simulink model "MotorModelContinuos"  (R2019b)
settings: Solver=VariableStepAuto  StartTime=0.0  StopTime=10  RelTol=1e-3
undefined symbols (not defined in the file or in its folder): C_max, I, I_max, J_m_star, k_t, L, P, R, tau_e, Ts
libraries: simulink x1
settings Model: Creator=AndreaCalegari  LastModifiedBy=AndreaCalegari

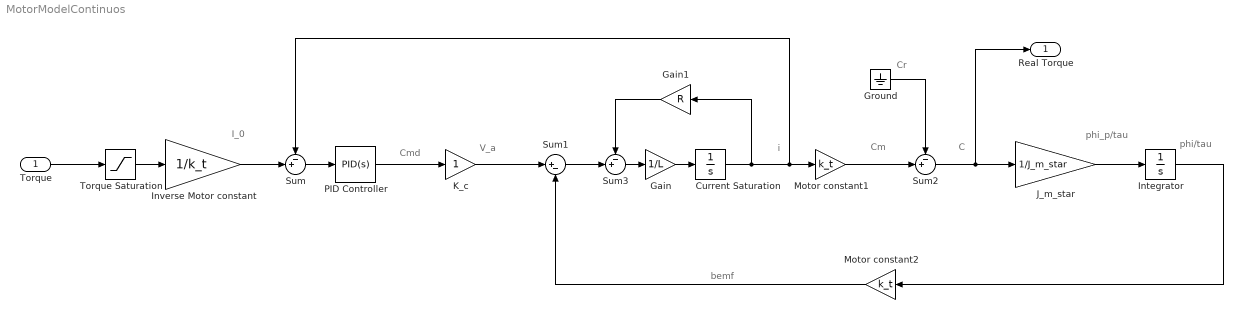
== system MotorModelContinuos ==
  note: i
  note: phi_p/tau
  note: I_0
  note: Cr
  note: bemf
  note: V_a
  note: C
  note: phi/tau
  note: Cmd
  note: Cm
  Torque : Inport  SampleTime=Ts
  Current Saturation : Integrator  LimitOutput=on  UpperSaturationLimit=I_max  LowerSaturationLimit=-I_max
  Gain : Gain  Gain=1/L
  Gain1 : Gain  Gain=R
  Ground : Ground
  Integrator : Integrator
  Inverse Motor constant : Gain  Gain=1/k_t
  "J_m_star " : Gain  Gain=1/J_m_star
  K_c : Gain
  Motor constant1 : Gain  Gain=k_t
  Motor constant2 : Gain  Gain=k_t
  PID Controller : simulink/Continuous/PID Controller  Controller=PID  Form=Parallel  TimeDomain=Continuous-time  SampleTime=-1  IntegratorMethod=Forward Euler  FilterMethod=Forward Euler  ControllerParametersSource=internal  P=P  I=I  D=0  UseFilter=on  N=100  TunerSelectOption=Transfer Function Based (PID Tuner App)  InitialConditionSource=internal  InitialConditionForIntegrator=0  InitialConditionForFilter=0  DifferentiatorICPrevScaledInput=0  ExternalReset=none  TrackingMode=off  Kt=1/tau_e  LimitOutput=off  UpperSaturationLimit=400  LowerSaturationLimit=-400  LinearizeAsGain=off  AntiWindupMode=clamping  Kb=1  POutMin=[]  POutMax=[]  IOutMin=[]  IOutMax=[]  DOutMin=[]  DOutMax=[]  NOutMin=[]  NOutMax=[]  SumOutMin=[]  SumOutMax=[]  SaturationOutMin=[]  SaturationOutMax=[]  PParamMin=[]  PParamMax=[]  IParamMin=[]  IParamMax=[]  DParamMin=[]  DParamMax=[]  NParamMin=[]  NParamMax=[]  KbParamMin=[]  KbParamMax=[]  KtParamMin=[]  KtParamMax=[]  KbOutMin=[]  KbOutMax=[]  KtOutMin=[]  KtOutMax=[]  IntegratorOutMin=[]  IntegratorOutMax=[]  FilterOutMin=[]  FilterOutMax=[]  SumI1OutMin=[]  SumI1OutMax=[]  SumI2OutMin=[]  SumI2OutMax=[]  SumI3OutMin=[]  SumI3OutMax=[]  SumI4OutMin=[]  SumI4OutMax=[]  SumDOutMin=[]  SumDOutMax=[]  DifferentiatorOutMin=[]  DifferentiatorOutMax=[]  FilterDiffOutCoefMin=[]  FilterDiffOutCoefMax=[]  ReciprocalOutMin=[]  ReciprocalOutMax=[]  SumDenOutMin=[]  SumDenOutMax=[]  SumNumOutMin=[]  SumNumOutMax=[]  DivideOutMin=[]  DivideOutMax=[]  IntegratorContinuousStateAttributes=''  IntegratorStateMustResolveToSignalObject=off  IntegratorRTWStateStorageClass=Auto  FilterContinuousStateAttributes=''  FilterStateMustResolveToSignalObject=off  FilterRTWStateStorageClass=Auto  ParallelPVariant=InternalParameters  IdealPVariant=Disabled  IVariant=InternalParameters  DVariant=InternalParameters  IntegratorVariant=Continuous  SatVariant=Disabled  AWVariant=Passthrough  PCopyVariant=Disabled  TRVariant=Disabled  FdbkBlocksVariant=Forward  IdealPFdbkVariant=Disabled  SatFdbkVariant=Disabled  DerivativeFilterVariant=ContFilter  NVariant=InternalParameters  NCopyVariant=Disabled  FilterICVariant=InternalICsFilter  IntegratorICVariant=InternalICs  ExternalResetVariant=Disabled  TRSumVariant=Passthrough  SumFdbkVariant=Disabled  SumVariant=Sum_PID
  Sum : Sum  Inputs=-+|
  Sum1 : Sum  Inputs=|+-
  Sum2 : Sum  Inputs=-+|
  Sum3 : Sum  Inputs=-+|
  Torque Saturation : Saturate  UpperLimit=C_max  LowerLimit=-C_max
  "Real Torque " : Outport
  wires:
  PID Controller/1 -> K_c/1
  Gain1/1 -> Sum3/1
  Sum/1 -> PID Controller/1
  Sum3/1 -> Gain/1
  Motor constant1/1 -> Sum2/2
  Ground/1 -> Sum2/1
  Current Saturation/1 -> Gain1/1, Sum/1, Motor constant1/1
  "J_m_star "/1 -> Integrator/1
  Gain/1 -> Current Saturation/1
  Torque/1 -> Torque Saturation/1
  Motor constant2/1 -> Sum1/2
  Sum1/1 -> Sum3/2
  K_c/1 -> Sum1/1
  Integrator/1 -> Motor constant2/1
  Inverse Motor constant/1 -> Sum/2
  Torque Saturation/1 -> Inverse Motor constant/1
  Sum2/1 -> "Real Torque "/1, "J_m_star "/1
